simulink model "City_Env_2Car_CS2020"  (Simulink 8.1)
settings: Solver=ode45  StartTime=0  StopTime=20  RelTol=1e-3
libraries: Solver_SF x2
settings Model: Creator=dhall  LastModifiedBy=elowe  ExtModeTrigMode=oneshot  ExtModeArmWhenConnect=off
settings DataIOCC: LimitDataPoints=off  SignalLoggingName=sigsOut
settings OptimizationCC: BooleanDataType=off  ExpressionDepthLimit=128  LocalBlockOutputs=off  InitFltsAndDblsToZero=on
settings DebuggingCC: SaveWithParameterizedLinksMsg=none  SignalResolutionControl=TryResolveAllWithWarning  SolverPrmCheckMsg=none  MultiTaskDSMMsg=warning  MultiTaskCondExecSysMsg=none  FcnCallInpInsideContextMsg=EnableAllAsWarning  FrameProcessingCompatibilityMsg=error
settings HardwareCC: TargetUnknown=on
settings GRTTargetCC: TargetFcnLib=ansi_tfl_tmw.mat  CodeReplacementLibrary=C89/C90 (ANSI)  CompOptLevelCompliant=off

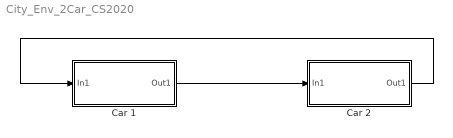
== system City_Env_2Car_CS2020 ==
  Car 1 : Subsystem
  Car 2 : Subsystem
  wires:
  Car 1/1(Out1) -> Car 2/1(In1)
  Car 2/1(Out1) -> Car 1/1(In1)

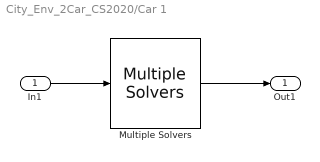
== system City_Env_2Car_CS2020/Car 1 ==
  In1 : Inport
  Multiple Solvers : Solver_SF/Multiple Solvers  Priority=1  iVehicle=1  SIMFILE=D:\mech_sim\trunk\Image\CarSim\Core\CarSim_Data\Extensions\Simulink\Multi_Vehicle\simfile1.sim  Run_RTs=off  vs_state_ind=Run  StopMode_ind=Vehicle Model  vs_scx=on
  Out1 : Outport
  wires:
  In1/1 -> Multiple Solvers/1
  Multiple Solvers/1 -> Out1/1

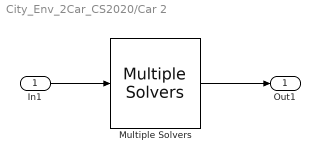
== system City_Env_2Car_CS2020/Car 2 ==
  In1 : Inport
  Multiple Solvers : Solver_SF/Multiple Solvers  Priority=1  iVehicle=2  SIMFILE=D:\mech_sim\trunk\Image\CarSim\Core\CarSim_Data\Extensions\Simulink\Multi_Vehicle\simfile2.sim  Run_RTs=off  vs_state_ind=Run  StopMode_ind=Vehicle Model  vs_scx=on
  Out1 : Outport
  wires:
  In1/1 -> Multiple Solvers/1
  Multiple Solvers/1 -> Out1/1
